simulink model "pendlib"  (Simulink 7.4)
settings: Solver=ode45  StartTime=0.0  StopTime=10.0  RelTol=1e-3
values from neighbouring files (symbols this model uses):
  Fscomp_neg = 0.16    [pendinit.m]
  Fscomp_pos = 0.16    [pendinit.m]
  g = 9.81    [pendinit.m]
  h = 0.01    [pendinit.m]
  J = 0.05    [pendinit.m]
  Jp = 0.0009    [pendinit.m]
  k1 = 0.058    [pendinit.m]
  k2 = 0.68    [pendinit.m]
  k360 = 0.3091    [pendinit.m]
  k4r = 2.56    [pendinit.m]
  k5r = 2.0    (= 2)    [pendinit.m]
  kdot360 = 3.76    [pendinit.m]
  ku = 1.40    (= 1.4)    [pendinit.m]
  l = l + 1    (= 1)    [asdf.m]    (also in pendinit.m = 0.413)
  M = 0.01    [pendinit.m]
  m = 0.02    [pendinit.m]
  offs1 = 0.7792    [pendinit.m]
  offs2 = 0    [pendinit.m]
  offs360 = 5.1763    [pendinit.m]
  offs4r = 0    [pendinit.m]
  offs5r = 0.0708    [pendinit.m]
  offsdot360 = -0.022    [pendinit.m]
  r = 0.235    [pendinit.m]
  w0 = 5.58    [pendinit.m]
  x0 = [0.1 0 0 0]'    [pendinit.m]
undefined symbols (not defined in the file or in its folder): DiscIntNeverNeededParam
libraries: simulink3 x5
settings Model: Creator=lincoln  LastModifiedBy=karl  ExtModeTrigMode=oneshot  ExtModeArmWhenConnect=off  ExtModeAutoUpdateStatusClock=off
settings DataIOCC: LimitDataPoints=off
settings OptimizationCC: BooleanDataType=off  InitFltsAndDblsToZero=on
settings DebuggingCC: SaveWithParameterizedLinksMsg=none  SignalResolutionControl=TryResolveAllWithWarning  SolverPrmCheckMsg=none  MultiTaskDSMMsg=warning  MultiTaskCondExecSysMsg=none  StrictBusMsg=None
settings HardwareCC: TargetUnknown=on
settings RTWCC: IncludeERTFirstTime=on
settings GRTTargetCC: TargetFcnLib=ansi_tfl_tmw.mat

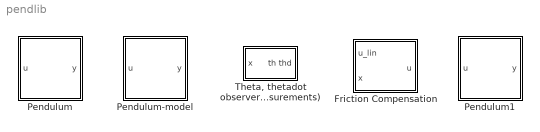
== system pendlib ==
  Friction Compensation : Subsystem  mask{khat=0}
      mask prompts: khat "k_hat"
  Pendulum : Subsystem
      mask Display: disp('Hardware')
  Pendulum-model : Subsystem
      mask Display: disp('Model')
  Pendulum1 : Subsystem
      mask Display: disp('Hardware\n Lab 2 Nonlin')
  "Theta, thetadot observer (for full 360 measurements)" : Subsystem

== system pendlib/Friction Compensation ==
  u_lin : Inport
  x : Inport  Port=2
  Friction model : Subsystem
  Selector : Selector  InputPortWidth=4  IndexOptions=Index vector (dialog)  Indices=4  OutputSizes=1
  u : Outport
  wires:
  Selector/1 -> Friction model/2(phidot)
  x/1 -> Selector/1
  u_lin/1 -> Friction model/1(u)
  Friction model/1(u_) -> u/1

== system pendlib/Pendulum ==
  u : Inport
  Hardware : Subsystem
  Safety net (switch off) : Subsystem
  Terminator : Terminator
  y : Outport  InitialOutput=0
  tag scope: u=global
  wires:
  Hardware/1(y) -> y/1
  Safety net (switch off)/1(u_out) -> [u], Hardware/1(u)
  u/1 -> Safety net (switch off)/1(u_in)
  [u] -> Terminator/1

== system pendlib/Pendulum-model ==
  u : Inport
  Pendulum Model : Subsystem
  Saturation : Saturate  UpperLimit=2  LowerLimit=-2
  Terminator : Terminator
  y : Outport  InitialOutput=0
  tag scope: u=global
  wires:
  Pendulum Model/1(x) -> y/1
  [u] -> Terminator/1
  u/1 -> Saturation/1
  Saturation/1 -> [u], Pendulum Model/1(u)

== system pendlib/Pendulum1 ==
  u : Inport
  Hardware : Subsystem
  Safety net (switch off) : Subsystem
  Terminator : Terminator
  y : Outport  InitialOutput=0
  tag scope: u=global
  wires:
  Hardware/1(y) -> y/1
  Safety net (switch off)/1(u_out) -> [u], Hardware/1(u)
  u/1 -> Safety net (switch off)/1(u_in)
  [u] -> Terminator/1

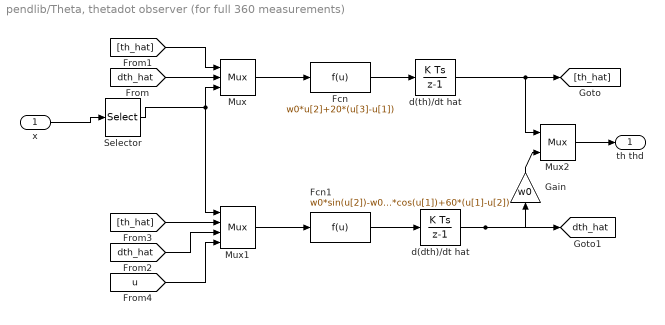
== system pendlib/Theta, thetadot observer (for full 360 measurements) ==
  x : Inport
  Fcn : Fcn  Expr=w0*u[2]+20*(u[3]-u[1])
  Fcn1 : Fcn  Expr=w0*sin(u[2])-w0*u[4]/g*cos(u[1])+60*(u[1]-u[2])
  Gain : Gain  Gain=w0  SaturateOnIntegerOverflow=on  OutDataTypeStr=Inherit: Same as input  ParamDataTypeStr=Inherit: Same as input
  Mux : Mux  Inputs=3
  Mux1 : Mux
  Mux2 : Mux  Inputs=2
  Selector : Selector  InputPortWidth=4  IndexOptions=Index vector (dialog)  Indices=1  OutputSizes=1
  d(dth)/dt hat : DiscreteIntegrator  SampleTime=h  ICPrevOutput=DiscIntNeverNeededParam  ICPrevScaledInput=DiscIntNeverNeededParam
  d(th)/dt hat : DiscreteIntegrator  InitialCondition=pi  SampleTime=h  ICPrevOutput=DiscIntNeverNeededParam  ICPrevScaledInput=DiscIntNeverNeededParam
  th thd : Outport
  tag scope: dth_hat=global
  wires:
  Mux/1 -> Fcn/1
  x/1 -> Selector/1
  Gain/1 -> Mux2/2
  d(dth)/dt hat/1 -> Gain/1, [dth_hat]
  [u] -> Mux1/4
  Fcn1/1 -> d(dth)/dt hat/1
  d(th)/dt hat/1 -> Mux2/1, [th_hat]
  Fcn/1 -> d(th)/dt hat/1
  [dth_hat] -> Mux1/3
  [th_hat] -> Mux1/2
  Mux1/1 -> Fcn1/1
  Mux2/1 -> th thd/1
  [dth_hat] -> Mux/2
  [th_hat] -> Mux/1
  Selector/1 -> Mux/3, Mux1/1

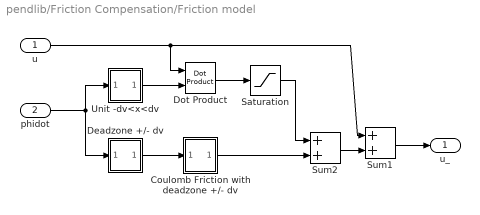
== system pendlib/Friction Compensation/Friction model ==
  u : Inport
  phidot : Inport  Port=2
  Coulomb Friction with deadzone +/- dv : Subsystem  mask{Fc_neg=khat, Fc_pos=khat, dv=0.06}
      mask prompts: Fc_neg "Coulomb Friction (Negative)"; Fc_pos "Coulomb Friction (Positive)"; dv "Deadzone width (Onesided)"
      mask Display:
      | plot([-1 0 0], [0 0 1], [0 0 1],[-1 0 0]);
      | plot([0.5 0.5 1],[0 0.5 0.5],[-0.5 -0.5 -1],[0 -0.5 -0.5]);
  Deadzone +/- dv : Subsystem  mask{vg=1, dv=0.06}
      mask prompts: vg "Gain"; dv "Deadzone width (Onesided)"
      mask init:
      | v_gain=vg;
      | d_v=dv;
      mask Display:
      | plot([-1 0 0], [0 0 1], [0 0 1],[-1 0 0]);
      | plot([0.5 0.5 1],[0 0.5 1],[-0.5 -0.5 -1],[0 -0.5 -1]);
  Dot Product : simulink3/Math/Dot Product  InputSameDT=on  DoSatur=off
  Saturation : Saturate  UpperLimit=khat  LowerLimit=-khat
  Sum1 : Sum  SaturateOnIntegerOverflow=on  InputSameDT=on  OutDataTypeStr=Inherit: Same as first input
  Sum2 : Sum  SaturateOnIntegerOverflow=on  InputSameDT=on  OutDataTypeStr=Inherit: Same as first input
  "Unit -dv<x<dv\t" : Subsystem  mask{dw=0.06}
      mask prompts: dw "Width (Onesided)"
      mask init:
      | d_w=dw;
      mask Display:
      | plot([-1 0 0], [0 0 1], [0 0 1],[-0.3 0 0]);
      | plot([-0.5 -0.5 0.5 0.5],[0 0.7 0.7 0])
  u_ : Outport  InitialOutput=0
  wires:
  phidot/1 -> "Unit -dv<x<dv\t"/1(In1), Deadzone +/- dv/1(In1)
  "Unit -dv<x<dv\t"/1(Out1) -> Dot Product/2
  Coulomb Friction with deadzone +/- dv/1(Out1) -> Sum2/2
  Dot Product/1 -> Saturation/1
  u/1 -> Dot Product/1, Sum1/1
  Saturation/1 -> Sum2/1
  Sum1/1 -> u_/1
  Deadzone +/- dv/1(Out1) -> Coulomb Friction with deadzone +/- dv/1(In1)
  Sum2/1 -> Sum1/2

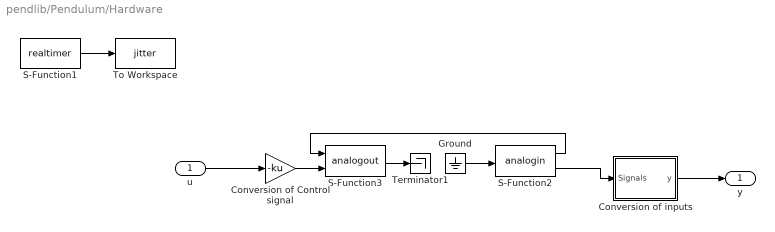
== system pendlib/Pendulum/Hardware ==
  u : Inport
  Conversion of Control signal : Gain  Gain=-ku  SaturateOnIntegerOverflow=on  OutDataTypeStr=Inherit: Same as input  ParamDataTypeStr=Inherit: Same as input
  Conversion of inputs : Subsystem
  Ground : Ground
  S-Function1 : S-Function  FunctionName=realtimer  Parameters=h  EnableBusSupport=off
  S-Function2 : S-Function  FunctionName=analogin  Parameters=h [0 0 1 1 2 2 3 3 4 4 5 5 6 6 7 7]  EnableBusSupport=off
  S-Function3 : S-Function  FunctionName=analogout  Parameters=h [0]  EnableBusSupport=off
  Terminator1 : Terminator
  To Workspace : ToWorkspace  VariableName=jitter  SampleTime=-1  SaveFormat=Array
  y : Outport
  wires:
  u/1 -> Conversion of Control signal/1
  Ground/1 -> S-Function2/1
  S-Function2/2 -> Conversion of inputs/1(Signals)
  S-Function3/1 -> Terminator1/1
  S-Function2/1 -> S-Function3/1
  Conversion of Control signal/1 -> S-Function3/2
  S-Function1/1 -> To Workspace/1
  Conversion of inputs/1(y) -> y/1

== system pendlib/Pendulum/Safety net (switch off) ==
  u_in : Inport
  Abs : Abs  SaturateOnIntegerOverflow=on
  Constant : Constant  Value=0
  Discrete Transfer Fcn : DiscreteTransferFcn  Numerator=[0.1]  Denominator=[1 -0.9]  SampleTime=h
  Relay : Relay  OnSwitchValue=3  OffSwitchValue=2
  Saturation1 : Saturate  UpperLimit=2  LowerLimit=-2
  Stop Simulation : Stop
  Switch : Switch  Threshold=0.5  SaturateOnIntegerOverflow=on  InputSameDT=on
  u_out : Outport
  wires:
  Discrete Transfer Fcn/1 -> Relay/1
  Relay/1 -> Stop Simulation/1, Switch/2
  Constant/1 -> Switch/1
  Abs/1 -> Discrete Transfer Fcn/1
  Switch/1 -> Saturation1/1
  Saturation1/1 -> u_out/1
  u_in/1 -> Switch/3, Abs/1

== system pendlib/Pendulum-model/Pendulum Model ==
  u : Inport
  "Friction Model Coulomb, Stic." : Subsystem
  Furuta pendulum : Subsystem  mask{l=l, M=M, Jp=Jp, r=r, J=J, m_w=m, g=g, x_0=x0}
      mask prompts: l "Pendulum Length"; M "Mass of Pendulum"; r "Length of Arm"; m_w "Mass of weight"
  Gain : Gain  Gain=g  SaturateOnIntegerOverflow=on  OutDataTypeStr=Inherit: Same as input  ParamDataTypeStr=Inherit: Same as input
  Sampling : Subsystem
  top-360 switching : Subsystem
  x : Outport  InitialOutput=0
  tag scope: phidot=global
  wires:
  top-360 switching/1(y_) -> x/1
  Sampling/1(x) -> top-360 switching/1(y)
  Furuta pendulum/1(angle) -> Sampling/1(Theta)
  Furuta pendulum/3(arm. ang.) -> Sampling/3(Phi)
  Furuta pendulum/2(angle vel.) -> Sampling/2(Thetadot)
  Furuta pendulum/4(arm. ang. vel.) -> Sampling/4(Phidot), [phidot]
  u/1 -> "Friction Model Coulomb, Stic."/1(u_)
  "Friction Model Coulomb, Stic."/1(u) -> Gain/1
  Gain/1 -> Furuta pendulum/1(u)

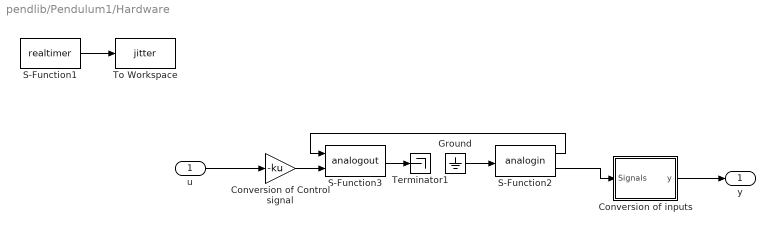
== system pendlib/Pendulum1/Hardware ==
  u : Inport
  Conversion of Control signal : Gain  Gain=-ku  SaturateOnIntegerOverflow=on  OutDataTypeStr=Inherit: Same as input  ParamDataTypeStr=Inherit: Same as input
  Conversion of inputs : Subsystem
  Ground : Ground
  S-Function1 : S-Function  FunctionName=realtimer  Parameters=h  EnableBusSupport=off
  S-Function2 : S-Function  FunctionName=analogin  Parameters=h [0 0 1 1 2 2 3 3 4 4 5 5 6 6 7 7]  EnableBusSupport=off
  S-Function3 : S-Function  FunctionName=analogout  Parameters=h [0]  EnableBusSupport=off
  Terminator1 : Terminator
  To Workspace : ToWorkspace  VariableName=jitter  SampleTime=-1  SaveFormat=Array
  y : Outport
  wires:
  u/1 -> Conversion of Control signal/1
  Ground/1 -> S-Function2/1
  S-Function2/2 -> Conversion of inputs/1(Signals)
  S-Function3/1 -> Terminator1/1
  S-Function2/1 -> S-Function3/1
  Conversion of Control signal/1 -> S-Function3/2
  S-Function1/1 -> To Workspace/1
  Conversion of inputs/1(y) -> y/1

== system pendlib/Pendulum1/Safety net (switch off) ==
  u_in : Inport
  Abs : Abs  SaturateOnIntegerOverflow=on
  Constant : Constant  Value=0
  Discrete Transfer Fcn : DiscreteTransferFcn  Numerator=[0.1]  Denominator=[1 -0.9]  SampleTime=h
  Relay : Relay  OnSwitchValue=3  OffSwitchValue=2
  Saturation1 : Saturate  UpperLimit=2  LowerLimit=-2
  Stop Simulation : Stop
  Switch : Switch  Threshold=0.5  SaturateOnIntegerOverflow=on  InputSameDT=on
  u_out : Outport
  wires:
  Discrete Transfer Fcn/1 -> Relay/1
  Relay/1 -> Stop Simulation/1, Switch/2
  Constant/1 -> Switch/1
  Abs/1 -> Discrete Transfer Fcn/1
  Switch/1 -> Saturation1/1
  Saturation1/1 -> u_out/1
  u_in/1 -> Switch/3, Abs/1

== system pendlib/Friction Compensation/Friction model/Coulomb Friction with deadzone +/- dv ==
  In1 : Inport
  Dead Zone : DeadZone  LowerValue=-dv  UpperValue=dv  SaturateOnIntegerOverflow=on
  Fcn : Fcn  Expr=(u<0)*u*Fc_neg+(u>0)*u*Fc_pos
  Sign : Signum
  Out1 : Outport  InitialOutput=0
  wires:
  Fcn/1 -> Out1/1
  Sign/1 -> Fcn/1
  Dead Zone/1 -> Sign/1
  In1/1 -> Dead Zone/1

== system pendlib/Friction Compensation/Friction model/Deadzone +/- dv ==
  In1 : Inport
  Constant : Constant  Value=d_v
  Dead Zone : DeadZone  LowerValue=-d_v  UpperValue=d_v  SaturateOnIntegerOverflow=on
  Dot Product : simulink3/Math/Dot Product  InputSameDT=on  DoSatur=off
  Gain : Gain  Gain=v_gain  SaturateOnIntegerOverflow=on  OutDataTypeStr=Inherit: Same as input  ParamDataTypeStr=Inherit: Same as input
  Sign : Signum
  Sum : Sum  SaturateOnIntegerOverflow=on  InputSameDT=on  OutDataTypeStr=Inherit: Same as first input
  Out1 : Outport  InitialOutput=0
  wires:
  Gain/1 -> Sum/1
  In1/1 -> Dead Zone/1
  Sign/1 -> Dot Product/1
  Dead Zone/1 -> Gain/1, Sign/1
  Constant/1 -> Dot Product/2
  Dot Product/1 -> Sum/2
  Sum/1 -> Out1/1

== system pendlib/Friction Compensation/Friction model/Unit -dv<x<dv	 ==
  In1 : Inport
  Abs : Abs  SaturateOnIntegerOverflow=on
  Constant : Constant
  Dead Zone : DeadZone  LowerValue=-d_w  UpperValue=d_w  SaturateOnIntegerOverflow=on
  Sign : Signum
  Sum1 : Sum  Inputs=+-  SaturateOnIntegerOverflow=on  InputSameDT=on  OutDataTypeStr=Inherit: Same as first input
  Out1 : Outport  InitialOutput=0
  wires:
  Dead Zone/1 -> Sign/1
  In1/1 -> Dead Zone/1
  Constant/1 -> Sum1/1
  Sum1/1 -> Out1/1
  Sign/1 -> Abs/1
  Abs/1 -> Sum1/2

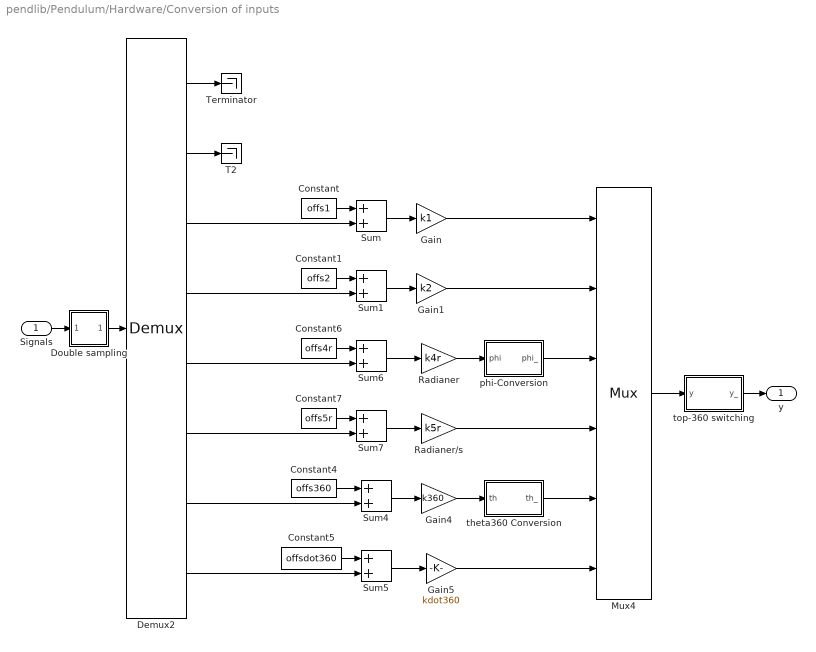
== system pendlib/Pendulum/Hardware/Conversion of inputs ==
  Signals : Inport
  Constant : Constant  Value=offs1
  Constant1 : Constant  Value=offs2
  Constant4 : Constant  Value=offs360
  Constant5 : Constant  Value=offsdot360
  Constant6 : Constant  Value=offs4r
  Constant7 : Constant  Value=offs5r
  Demux2 : Demux  Outputs=8
  Double sampling : Subsystem
  Gain : Gain  Gain=k1  SaturateOnIntegerOverflow=on  OutDataTypeStr=Inherit: Same as input  ParamDataTypeStr=Inherit: Same as input
  Gain1 : Gain  Gain=k2  SaturateOnIntegerOverflow=on  OutDataTypeStr=Inherit: Same as input  ParamDataTypeStr=Inherit: Same as input
  Gain4 : Gain  Gain=k360  SaturateOnIntegerOverflow=on  OutDataTypeStr=Inherit: Same as input  ParamDataTypeStr=Inherit: Same as input
  Gain5 : Gain  Gain=kdot360  SaturateOnIntegerOverflow=on  OutDataTypeStr=Inherit: Same as input  ParamDataTypeStr=Inherit: Same as input
  Mux4 : Mux  Inputs=6
  Radianer : Gain  Gain=k4r  SaturateOnIntegerOverflow=on  OutDataTypeStr=Inherit: Same as input  ParamDataTypeStr=Inherit: Same as input
  Radianer/s : Gain  Gain=k5r  SaturateOnIntegerOverflow=on  OutDataTypeStr=Inherit: Same as input  ParamDataTypeStr=Inherit: Same as input
  Sum{,1,4..7} (6 alike) : Sum  SaturateOnIntegerOverflow=on  InputSameDT=on  OutDataTypeStr=Inherit: Same as first input
  T2 : Terminator
  Terminator : Terminator
  phi-Conversion : Subsystem
  theta360 Conversion : Subsystem
  top-360 switching : Subsystem
  y : Outport  InitialOutput=0
  wires:
  Demux2/2 -> T2/1
  Demux2/1 -> Terminator/1
  Sum/1 -> Gain/1
  Constant/1 -> Sum/1
  Sum1/1 -> Gain1/1
  Constant1/1 -> Sum1/1
  Sum4/1 -> Gain4/1
  Sum5/1 -> Gain5/1
  Constant5/1 -> Sum5/1
  Sum6/1 -> Radianer/1
  Constant6/1 -> Sum6/1
  Radianer/1 -> phi-Conversion/1(phi)
  Sum7/1 -> Radianer/s/1
  Constant7/1 -> Sum7/1
  Mux4/1 -> top-360 switching/1(y)
  top-360 switching/1(y_) -> y/1
  Constant4/1 -> Sum4/1
  Demux2/5 -> Sum6/2
  Demux2/6 -> Sum7/2
  phi-Conversion/1(phi_) -> Mux4/3
  Radianer/s/1 -> Mux4/4
  theta360 Conversion/1(th_) -> Mux4/5
  Signals/1 -> Double sampling/1(In1)
  Double sampling/1(Out1) -> Demux2/1
  Gain4/1 -> theta360 Conversion/1(th)
  Gain5/1 -> Mux4/6
  Gain/1 -> Mux4/1
  Demux2/3 -> Sum/2
  Demux2/4 -> Sum1/2
  Demux2/7 -> Sum4/2
  Demux2/8 -> Sum5/2
  Gain1/1 -> Mux4/2

== system pendlib/Pendulum-model/Pendulum Model/Friction Model Coulomb, Stic. ==
  u_ : Inport
  Friction model : Subsystem
  u : Outport  InitialOutput=0
  wires:
  Friction model/1(u_) -> u/1
  [phidot] -> Friction model/2(phidot)
  u_/1 -> Friction model/1(u)

== system pendlib/Pendulum-model/Pendulum Model/Furuta pendulum ==
  u : Inport
  Demux : Demux
  S-Function1 : S-Function  FunctionName=furuta  Parameters=l, M, Jp, r, J, m_w, g, x_0  EnableBusSupport=off
  angle : Outport  InitialOutput=0
  angle vel. : Outport  Port=2  InitialOutput=0
  arm. ang. : Outport  Port=3  InitialOutput=0
  arm. ang. vel. : Outport  Port=4  InitialOutput=0
  wires:
  Demux/4 -> arm. ang. vel./1
  Demux/3 -> arm. ang./1
  u/1 -> S-Function1/1
  Demux/2 -> angle vel./1
  Demux/1 -> angle/1
  S-Function1/1 -> Demux/1

== system pendlib/Pendulum-model/Pendulum Model/Sampling ==
  Theta : Inport
  Thetadot : Inport  Port=2
  Phi : Inport  Port=3
  Phidot : Inport  Port=4
  Demux : Demux  Outputs=[3 1]
  Mux : Mux
  Mux1 : Mux  Inputs=2
  Zero-Order Hold5 : ZeroOrderHold  SampleTime=h
  x : Outport  InitialOutput=0
  wires:
  Demux/2 -> Mux1/2
  Theta/1 -> Mux/1
  Thetadot/1 -> Mux/2
  Phi/1 -> Mux/3
  Phidot/1 -> Mux/4
  Mux/1 -> Zero-Order Hold5/1
  Zero-Order Hold5/1 -> Demux/1
  Mux1/1 -> x/1
  Demux/1 -> Mux1/1

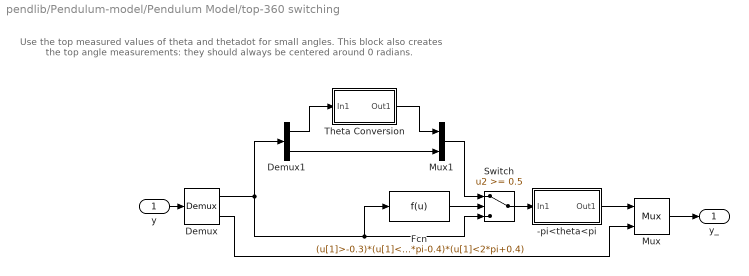
== system pendlib/Pendulum-model/Pendulum Model/top-360 switching ==
  note: Use the top measured values of
      | theta and thetadot for small angles.
      | This block also creates the top angle
      | measurements: they should always be
      | centered around 0 radians.
  y : Inport
  -pi<theta<pi : Subsystem
  Demux : Demux  Outputs=[2 2]
  Demux1 : Demux  Outputs=2
  Fcn : Fcn  Expr=(u[1]>-0.3)*(u[1]<0.4)+(u[1]>2*pi-0.4)*(u[1]<2*pi+0.4)
  Mux : Mux  Inputs=2
  Mux1 : Mux  Inputs=2
  Switch : Switch  Threshold=0.5  SaturateOnIntegerOverflow=on  InputSameDT=on
  Theta Conversion : Subsystem
  y_ : Outport
  wires:
  Mux1/1 -> Switch/1
  Demux1/2 -> Mux1/2
  Demux1/1 -> Theta Conversion/1(In1)
  Demux/1 -> Fcn/1, Switch/3, Demux1/1
  Demux/2 -> Mux/2
  y/1 -> Demux/1
  Mux/1 -> y_/1
  Fcn/1 -> Switch/2
  Theta Conversion/1(Out1) -> Mux1/1
  Switch/1 -> -pi<theta<pi/1(In1)
  -pi<theta<pi/1(Out1) -> Mux/1

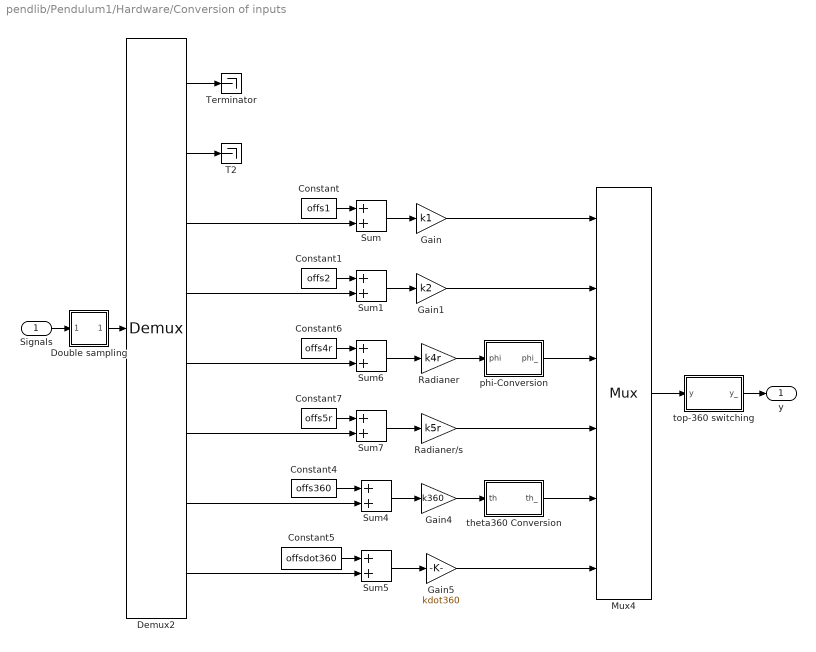
== system pendlib/Pendulum1/Hardware/Conversion of inputs ==
  Signals : Inport
  Constant : Constant  Value=offs1
  Constant1 : Constant  Value=offs2
  Constant4 : Constant  Value=offs360
  Constant5 : Constant  Value=offsdot360
  Constant6 : Constant  Value=offs4r
  Constant7 : Constant  Value=offs5r
  Demux2 : Demux  Outputs=8
  Double sampling : Subsystem
  Gain : Gain  Gain=k1  SaturateOnIntegerOverflow=on  OutDataTypeStr=Inherit: Same as input  ParamDataTypeStr=Inherit: Same as input
  Gain1 : Gain  Gain=k2  SaturateOnIntegerOverflow=on  OutDataTypeStr=Inherit: Same as input  ParamDataTypeStr=Inherit: Same as input
  Gain4 : Gain  Gain=k360  SaturateOnIntegerOverflow=on  OutDataTypeStr=Inherit: Same as input  ParamDataTypeStr=Inherit: Same as input
  Gain5 : Gain  Gain=kdot360  SaturateOnIntegerOverflow=on  OutDataTypeStr=Inherit: Same as input  ParamDataTypeStr=Inherit: Same as input
  Mux4 : Mux  Inputs=6
  Radianer : Gain  Gain=k4r  SaturateOnIntegerOverflow=on  OutDataTypeStr=Inherit: Same as input  ParamDataTypeStr=Inherit: Same as input
  Radianer/s : Gain  Gain=k5r  SaturateOnIntegerOverflow=on  OutDataTypeStr=Inherit: Same as input  ParamDataTypeStr=Inherit: Same as input
  Sum{,1,4..7} (6 alike) : Sum  SaturateOnIntegerOverflow=on  InputSameDT=on  OutDataTypeStr=Inherit: Same as first input
  T2 : Terminator
  Terminator : Terminator
  phi-Conversion : Subsystem
  theta360 Conversion : Subsystem
  top-360 switching : Subsystem
  y : Outport  InitialOutput=0
  wires:
  Demux2/2 -> T2/1
  Demux2/1 -> Terminator/1
  Sum/1 -> Gain/1
  Constant/1 -> Sum/1
  Sum1/1 -> Gain1/1
  Constant1/1 -> Sum1/1
  Sum4/1 -> Gain4/1
  Sum5/1 -> Gain5/1
  Constant5/1 -> Sum5/1
  Sum6/1 -> Radianer/1
  Constant6/1 -> Sum6/1
  Radianer/1 -> phi-Conversion/1(phi)
  Sum7/1 -> Radianer/s/1
  Constant7/1 -> Sum7/1
  Mux4/1 -> top-360 switching/1(y)
  top-360 switching/1(y_) -> y/1
  Constant4/1 -> Sum4/1
  Demux2/5 -> Sum6/2
  Demux2/6 -> Sum7/2
  phi-Conversion/1(phi_) -> Mux4/3
  Radianer/s/1 -> Mux4/4
  theta360 Conversion/1(th_) -> Mux4/5
  Signals/1 -> Double sampling/1(In1)
  Double sampling/1(Out1) -> Demux2/1
  Gain4/1 -> theta360 Conversion/1(th)
  Gain5/1 -> Mux4/6
  Gain/1 -> Mux4/1
  Demux2/3 -> Sum/2
  Demux2/4 -> Sum1/2
  Demux2/7 -> Sum4/2
  Demux2/8 -> Sum5/2
  Gain1/1 -> Mux4/2

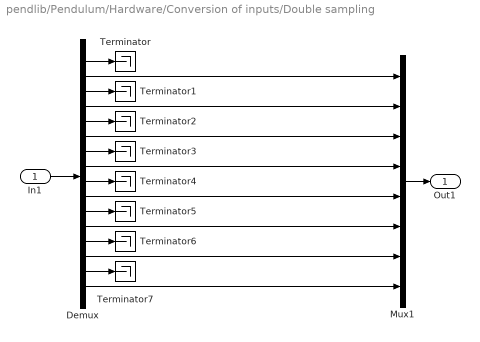
== system pendlib/Pendulum/Hardware/Conversion of inputs/Double sampling ==
  In1 : Inport
  Demux : Demux  Outputs=16
  Mux1 : Mux  Inputs=8
  Terminator{,1..7} (8 alike) : Terminator
  Out1 : Outport
  wires:
  Demux/7 -> Terminator3/1
  Demux/9 -> Terminator4/1
  Demux/11 -> Terminator5/1
  Demux/13 -> Terminator6/1
  Demux/15 -> Terminator7/1
  Demux/5 -> Terminator2/1
  Demux/3 -> Terminator1/1
  Demux/1 -> Terminator/1
  In1/1 -> Demux/1
  Demux/2 -> Mux1/1
  Mux1/1 -> Out1/1
  Demux/4 -> Mux1/2
  Demux/6 -> Mux1/3
  Demux/8 -> Mux1/4
  Demux/10 -> Mux1/5
  Demux/12 -> Mux1/6
  Demux/14 -> Mux1/7
  Demux/16 -> Mux1/8

== system pendlib/Pendulum/Hardware/Conversion of inputs/phi-Conversion ==
  note: This block deals with the discontinious nature
      | of the phi signal. The offset is kept in the integrator.
  phi : Inport
  Diff : DiscreteTransferFcn  Numerator=[1 -1]  Denominator=[1 0]  SampleTime=h
  Extended Deadzone : Subsystem  mask{vg=1, dv=0.5}
      mask prompts: vg "Gain"; dv "Deadzone width"
      mask init:
      | v_gain=vg;
      | d_v=dv;
      mask Display:
      | plot([-1 0 0], [0 0 1], [0 0 1],[-1 0 0]);
      | plot([0.5 0.5 1],[0 0.5 1],[-0.5 -0.5 -1],[0 -0.5 -1]);
  Gain1 : Gain  Gain=-1  SaturateOnIntegerOverflow=on  OutDataTypeStr=Inherit: Same as input  ParamDataTypeStr=Inherit: Same as input
  Integrate : DiscreteTransferFcn  Denominator=[1 -1]  SampleTime=h
  Sum2 : Sum  SaturateOnIntegerOverflow=on  InputSameDT=on  OutDataTypeStr=Inherit: Same as first input
  Sum3 : Sum  SaturateOnIntegerOverflow=on  InputSameDT=on  OutDataTypeStr=Inherit: Same as first input
  phi_ : Outport
  wires:
  Sum2/1 -> Gain1/1
  phi/1 -> Diff/1, Sum3/2
  Gain1/1 -> Sum3/1
  Integrate/1 -> Sum2/2
  Extended Deadzone/1(Out1) -> Integrate/1, Sum2/1
  Sum3/1 -> phi_/1
  Diff/1 -> Extended Deadzone/1(In1)

== system pendlib/Pendulum/Hardware/Conversion of inputs/theta360 Conversion ==
  note: The measure of Theta is discontinous and must hereby
      | be modifyed in order to give a reasonable continous signal.
  th : Inport
  Fcn : Fcn  Expr=((u[1]-u[2])>2)*(-2*pi)+((u[1]-u[2])<-2)*(2*pi)
  Last sample : UnitDelay  X0=pi  SampleTime=h
  Mux : Mux  Inputs=2
  Offset : Subsystem
  Scope2 : Scope
      settings: TimeRange=25  YMin=-0.4  YMax=0.05
  Spike Filter6 : Subsystem
  Sum3 : Sum  SaturateOnIntegerOverflow=on  InputSameDT=on  OutDataTypeStr=Inherit: Same as first input
  th_ : Outport
  wires:
  Mux/1 -> Fcn/1
  th/1 -> Last sample/1, Mux/1, Sum3/1
  Last sample/1 -> Mux/2
  Fcn/1 -> Offset/1(In1)
  Offset/1(Out1) -> Sum3/2
  Sum3/1 -> Spike Filter6/1(x)
  Spike Filter6/1(x_) -> th_/1, Scope2/1

== system pendlib/Pendulum/Hardware/Conversion of inputs/top-360 switching ==
  note: Use the top measured values of
      | theta and thetadot for small angles
  y : Inport
  Demux : Demux  Outputs=[2 2 2]
  Fcn : Fcn  Expr=(u[1]>-0.5)*(u[1]<0.5)+(u[1]>2*pi-0.5)*(u[1]<2*pi+0.5)
  Mux : Mux  Inputs=2
  Switch : Switch  Threshold=0.5  SaturateOnIntegerOverflow=on  InputSameDT=on
  y_ : Outport
  wires:
  y/1 -> Demux/1
  Demux/2 -> Mux/2
  Demux/1 -> Switch/1
  Demux/3 -> Switch/3, Fcn/1
  Switch/1 -> Mux/1
  Fcn/1 -> Switch/2
  Mux/1 -> y_/1

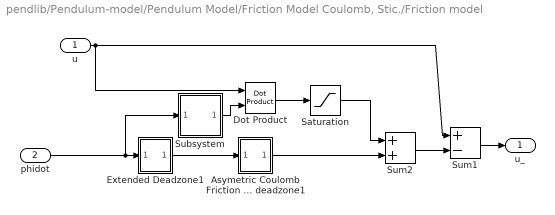
== system pendlib/Pendulum-model/Pendulum Model/Friction Model Coulomb, Stic./Friction model ==
  u : Inport
  phidot : Inport  Port=2
  Asymetric Coulomb Friction with deadzone1 : Subsystem  mask{Fc_neg=Fscomp_neg, Fc_pos=Fscomp_pos, dv=0.04}
      mask prompts: Fc_neg "Coulomb Friction (Negative)"; Fc_pos "Coulomb Friction (Positive)"; dv "Deadzone width (Onesided)"
      mask Display:
      | plot([-1 0 0], [0 0 1], [0 0 1],[-1 0 0]);
      | plot([0.5 0.5 1],[0 0.5 0.5],[-0.5 -0.5 -1],[0 -0.5 -0.5]);
  Dot Product : simulink3/Math/Dot Product  InputSameDT=on  DoSatur=off
  Extended Deadzone1 : Subsystem  mask{vg=1, dv=0.04}
      mask prompts: vg "Gain"; dv "Deadzone width (Onesided)"
      mask init:
      | v_gain=vg;
      | d_v=dv;
      mask Display:
      | plot([-1 0 0], [0 0 1], [0 0 1],[-1 0 0]);
      | plot([0.5 0.5 1],[0 0.5 1],[-0.5 -0.5 -1],[0 -0.5 -1]);
  Saturation : Saturate  UpperLimit=Fscomp_pos  LowerLimit=-Fscomp_neg
  Subsystem : Subsystem  mask{dw=0.04}
      mask prompts: dw "Width (Onesided)"
      mask init:
      | d_w=dw;
      mask Display:
      | plot([-1 0 0], [0 0 1], [0 0 1],[-0.3 0 0]);
      | plot([-0.5 -0.5 0.5 0.5],[0 0.7 0.7 0])
  Sum1 : Sum  Inputs=+-  SaturateOnIntegerOverflow=on  InputSameDT=on  OutDataTypeStr=Inherit: Same as first input
  Sum2 : Sum  SaturateOnIntegerOverflow=on  InputSameDT=on  OutDataTypeStr=Inherit: Same as first input
  u_ : Outport  InitialOutput=0
  wires:
  Asymetric Coulomb Friction with deadzone1/1(Out1) -> Sum2/2
  Sum2/1 -> Sum1/2
  u/1 -> Sum1/1, Dot Product/1
  Dot Product/1 -> Saturation/1
  Subsystem/1(Out1) -> Dot Product/2
  Extended Deadzone1/1(Out1) -> Asymetric Coulomb Friction with deadzone1/1(In1)
  Sum1/1 -> u_/1
  phidot/1 -> Subsystem/1(In1), Extended Deadzone1/1(In1)
  Saturation/1 -> Sum2/1

== system pendlib/Pendulum-model/Pendulum Model/top-360 switching/-pi<theta<pi ==
  In1 : Inport
  Constant : Constant  Value=2*pi
  Constant1 : Constant  Value=pi
  Demux : Demux  Outputs=2
  Math Function : Math  Operator=mod  SaturateOnIntegerOverflow=on
  Mux : Mux  Inputs=2
  Product : Product  SaturateOnIntegerOverflow=on  RndMeth=Zero  InputSameDT=on  OutDataTypeStr=Inherit: Same as first input
  Relational Operator : RelationalOperator  InputSameDT=on
  Sum : Sum  Inputs=|+-  SaturateOnIntegerOverflow=on  InputSameDT=on  OutDataTypeStr=Inherit: Same as first input
  Out1 : Outport
  wires:
  Constant/1 -> Math Function/2, Product/2
  Math Function/1 -> Sum/1, Relational Operator/1
  Constant1/1 -> Relational Operator/2
  Relational Operator/1 -> Product/1
  Product/1 -> Sum/2
  In1/1 -> Demux/1
  Demux/1 -> Math Function/1
  Sum/1 -> Mux/1
  Mux/1 -> Out1/1
  Demux/2 -> Mux/2

== system pendlib/Pendulum-model/Pendulum Model/top-360 switching/Theta Conversion ==
  In1 : Inport
  Fcn1 : Fcn  Expr=(u[1]-u[2])*2*pi-pi
  Fcn2 : Fcn  Expr=u/(2*pi)-1/2
  Mux : Mux  Inputs=2
  Rounding Function : Rounding
  Out1 : Outport  InitialOutput=0
  wires:
  Rounding Function/1 -> Mux/2
  Fcn2/1 -> Rounding Function/1, Mux/1
  Mux/1 -> Fcn1/1
  Fcn1/1 -> Out1/1
  In1/1 -> Fcn2/1

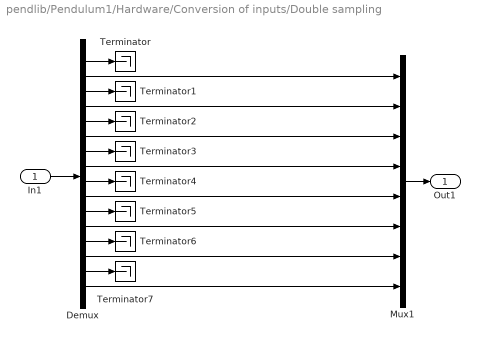
== system pendlib/Pendulum1/Hardware/Conversion of inputs/Double sampling ==
  In1 : Inport
  Demux : Demux  Outputs=16
  Mux1 : Mux  Inputs=8
  Terminator{,1..7} (8 alike) : Terminator
  Out1 : Outport
  wires:
  Demux/7 -> Terminator3/1
  Demux/9 -> Terminator4/1
  Demux/11 -> Terminator5/1
  Demux/13 -> Terminator6/1
  Demux/15 -> Terminator7/1
  Demux/5 -> Terminator2/1
  Demux/3 -> Terminator1/1
  Demux/1 -> Terminator/1
  In1/1 -> Demux/1
  Demux/2 -> Mux1/1
  Mux1/1 -> Out1/1
  Demux/4 -> Mux1/2
  Demux/6 -> Mux1/3
  Demux/8 -> Mux1/4
  Demux/10 -> Mux1/5
  Demux/12 -> Mux1/6
  Demux/14 -> Mux1/7
  Demux/16 -> Mux1/8

== system pendlib/Pendulum1/Hardware/Conversion of inputs/phi-Conversion ==
  note: This block deals with the discontinious nature
      | of the phi signal. The offset is kept in the integrator.
  phi : Inport
  Diff : DiscreteTransferFcn  Numerator=[1 -1]  Denominator=[1 0]  SampleTime=h
  Extended Deadzone : Subsystem  mask{vg=1, dv=0.5}
      mask prompts: vg "Gain"; dv "Deadzone width"
      mask init:
      | v_gain=vg;
      | d_v=dv;
      mask Display:
      | plot([-1 0 0], [0 0 1], [0 0 1],[-1 0 0]);
      | plot([0.5 0.5 1],[0 0.5 1],[-0.5 -0.5 -1],[0 -0.5 -1]);
  Gain1 : Gain  Gain=-1  SaturateOnIntegerOverflow=on  OutDataTypeStr=Inherit: Same as input  ParamDataTypeStr=Inherit: Same as input
  Integrate : DiscreteTransferFcn  Denominator=[1 -1]  SampleTime=h
  Sum2 : Sum  SaturateOnIntegerOverflow=on  InputSameDT=on  OutDataTypeStr=Inherit: Same as first input
  Sum3 : Sum  SaturateOnIntegerOverflow=on  InputSameDT=on  OutDataTypeStr=Inherit: Same as first input
  phi_ : Outport
  wires:
  Sum2/1 -> Gain1/1
  phi/1 -> Diff/1, Sum3/2
  Gain1/1 -> Sum3/1
  Integrate/1 -> Sum2/2
  Extended Deadzone/1(Out1) -> Integrate/1, Sum2/1
  Sum3/1 -> phi_/1
  Diff/1 -> Extended Deadzone/1(In1)

== system pendlib/Pendulum1/Hardware/Conversion of inputs/theta360 Conversion ==
  note: The measure of Theta is discontinous and must hereby
      | be modifyed in order to give a reasonable continous signal.
  th : Inport
  Fcn : Fcn  Expr=((u[1]-u[2])>2)*(-2*pi)+((u[1]-u[2])<-2)*(2*pi)
  Last sample : UnitDelay  X0=pi  SampleTime=h
  Mux : Mux  Inputs=2
  Offset : Subsystem
  Scope2 : Scope
      settings: TimeRange=25  YMin=-0.4  YMax=0.05
  Spike Filter6 : Subsystem
  Sum3 : Sum  SaturateOnIntegerOverflow=on  InputSameDT=on  OutDataTypeStr=Inherit: Same as first input
  th_ : Outport
  wires:
  Mux/1 -> Fcn/1
  th/1 -> Last sample/1, Mux/1, Sum3/1
  Last sample/1 -> Mux/2
  Fcn/1 -> Offset/1(In1)
  Offset/1(Out1) -> Sum3/2
  Sum3/1 -> Spike Filter6/1(x)
  Spike Filter6/1(x_) -> th_/1, Scope2/1

== system pendlib/Pendulum1/Hardware/Conversion of inputs/top-360 switching ==
  note: Use the top measured values of
      | theta and thetadot for small angles
  y : Inport
  Demux : Demux  Outputs=[2 2 2]
  Fcn : Fcn  Expr=(u[1]>-0.5)*(u[1]<0.5)+(u[1]>2*pi-0.5)*(u[1]<2*pi+0.5)
  ModTheta : Subsystem
  Mux : Mux  Inputs=2
  Scope1 : Scope
      settings: YMin=-4  YMax=7  SaveName=ScopeData3
  Switch : Switch  Threshold=0.5  SaturateOnIntegerOverflow=on  InputSameDT=on
  y_ : Outport
  wires:
  Switch/1 -> Mux/1
  ModTheta/1(xMod) -> Fcn/1, Switch/3
  Demux/3 -> ModTheta/1(x)
  y/1 -> Demux/1
  Demux/2 -> Mux/2
  Demux/1 -> Scope1/1, Switch/1
  Fcn/1 -> Switch/2
  Mux/1 -> y_/1

== system pendlib/Pendulum/Hardware/Conversion of inputs/phi-Conversion/Extended Deadzone ==
  In1 : Inport
  Constant : Constant  Value=d_v
  Dead Zone : DeadZone  LowerValue=-d_v  UpperValue=d_v  SaturateOnIntegerOverflow=on
  Dot Product : simulink3/Math/Dot Product  InputSameDT=on  DoSatur=off
  Gain : Gain  Gain=v_gain  SaturateOnIntegerOverflow=on  OutDataTypeStr=Inherit: Same as input  ParamDataTypeStr=Inherit: Same as input
  Sign : Signum
  Sum : Sum  SaturateOnIntegerOverflow=on  InputSameDT=on  OutDataTypeStr=Inherit: Same as first input
  Out1 : Outport  InitialOutput=0
  wires:
  Sum/1 -> Out1/1
  Dot Product/1 -> Sum/2
  Constant/1 -> Dot Product/2
  Dead Zone/1 -> Sign/1, Gain/1
  Sign/1 -> Dot Product/1
  In1/1 -> Dead Zone/1
  Gain/1 -> Sum/1

== system pendlib/Pendulum/Hardware/Conversion of inputs/theta360 Conversion/Offset ==
  note: Make sure only one
      | trig per lap.
  In1 : Inport
  Fcn : Fcn  Expr=(abs(u[1]+u[2])>8)*0+(abs(u[1]+u[2])<8)*u[1]
  Integrate : DiscreteTransferFcn  Denominator=[1 -1]  SampleTime=h
  Last offset : UnitDelay  X0=pi  SampleTime=h
  Mux : Mux  Inputs=2
  Out1 : Outport  InitialOutput=0
  wires:
  Mux/1 -> Fcn/1
  In1/1 -> Mux/1, Last offset/1
  Last offset/1 -> Mux/2
  Fcn/1 -> Integrate/1
  Integrate/1 -> Out1/1

== system pendlib/Pendulum/Hardware/Conversion of inputs/theta360 Conversion/Spike Filter6 ==
  x : Inport
  Fcn : Fcn  Expr=(abs(u[1]-u[2])<0.5)*u[1]+(abs(u[1]-u[2])>0.5)*u[3]
  Last Chosen : UnitDelay  X0=pi  SampleTime=h
  Last sample : UnitDelay  X0=pi  SampleTime=h
  Mux : Mux  Inputs=3
  Scope1 : Scope
      settings: YMin=0  YMax=11
  Scope2 : Scope
      settings: YMin=9  YMax=9.9
  x_ : Outport
  wires:
  Last Chosen/1 -> Mux/3
  Last sample/1 -> Mux/2
  x/1 -> Last sample/1, Mux/1
  Fcn/1 -> x_/1, Scope1/1, Last Chosen/1
  Mux/1 -> Fcn/1, Scope2/1

== system pendlib/Pendulum-model/Pendulum Model/Friction Model Coulomb, Stic./Friction model/Asymetric Coulomb Friction with deadzone1 ==
  In1 : Inport
  Dead Zone : DeadZone  LowerValue=-dv  UpperValue=dv  SaturateOnIntegerOverflow=on
  Fcn : Fcn  Expr=(u<0)*u*Fc_neg+(u>0)*u*Fc_pos
  Sign : Signum
  Out1 : Outport  InitialOutput=0
  wires:
  In1/1 -> Dead Zone/1
  Dead Zone/1 -> Sign/1
  Sign/1 -> Fcn/1
  Fcn/1 -> Out1/1

== system pendlib/Pendulum-model/Pendulum Model/Friction Model Coulomb, Stic./Friction model/Extended Deadzone1 ==
  In1 : Inport
  Constant : Constant  Value=d_v
  Dead Zone : DeadZone  LowerValue=-d_v  UpperValue=d_v  SaturateOnIntegerOverflow=on
  Dot Product : simulink3/Math/Dot Product  InputSameDT=on  DoSatur=off
  Gain : Gain  Gain=v_gain  SaturateOnIntegerOverflow=on  OutDataTypeStr=Inherit: Same as input  ParamDataTypeStr=Inherit: Same as input
  Sign : Signum
  Sum : Sum  SaturateOnIntegerOverflow=on  InputSameDT=on  OutDataTypeStr=Inherit: Same as first input
  Out1 : Outport  InitialOutput=0
  wires:
  Sum/1 -> Out1/1
  Dot Product/1 -> Sum/2
  Constant/1 -> Dot Product/2
  Dead Zone/1 -> Sign/1, Gain/1
  Sign/1 -> Dot Product/1
  In1/1 -> Dead Zone/1
  Gain/1 -> Sum/1

== system pendlib/Pendulum-model/Pendulum Model/Friction Model Coulomb, Stic./Friction model/Subsystem ==
  In1 : Inport
  Abs : Abs  SaturateOnIntegerOverflow=on
  Constant : Constant
  Dead Zone : DeadZone  LowerValue=-d_w  UpperValue=d_w  SaturateOnIntegerOverflow=on
  Sign : Signum
  Sum1 : Sum  Inputs=+-  SaturateOnIntegerOverflow=on  InputSameDT=on  OutDataTypeStr=Inherit: Same as first input
  Out1 : Outport  InitialOutput=0
  wires:
  Abs/1 -> Sum1/2
  Sign/1 -> Abs/1
  Sum1/1 -> Out1/1
  Constant/1 -> Sum1/1
  In1/1 -> Dead Zone/1
  Dead Zone/1 -> Sign/1

== system pendlib/Pendulum1/Hardware/Conversion of inputs/phi-Conversion/Extended Deadzone ==
  In1 : Inport
  Constant : Constant  Value=d_v
  Dead Zone : DeadZone  LowerValue=-d_v  UpperValue=d_v  SaturateOnIntegerOverflow=on
  Dot Product : DotProduct  OutDataType=fixdt(1, 16)  OutScaling=2^-10  InputSameDT=on  OutDataTypeStr=Inherit: Inherit via internal rule
  Gain : Gain  Gain=v_gain  SaturateOnIntegerOverflow=on  OutDataTypeStr=Inherit: Same as input  ParamDataTypeStr=Inherit: Same as input
  Sign : Signum
  Sum : Sum  SaturateOnIntegerOverflow=on  InputSameDT=on  OutDataTypeStr=Inherit: Same as first input
  Out1 : Outport  InitialOutput=0
  wires:
  Sum/1 -> Out1/1
  Dot Product/1 -> Sum/2
  Constant/1 -> Dot Product/2
  Dead Zone/1 -> Sign/1, Gain/1
  Sign/1 -> Dot Product/1
  In1/1 -> Dead Zone/1
  Gain/1 -> Sum/1

== system pendlib/Pendulum1/Hardware/Conversion of inputs/theta360 Conversion/Offset ==
  note: Make sure only one
      | trig per lap.
  In1 : Inport
  Fcn : Fcn  Expr=(abs(u[1]+u[2])>8)*0+(abs(u[1]+u[2])<8)*u[1]
  Integrate : DiscreteTransferFcn  Denominator=[1 -1]  SampleTime=h
  Last offset : UnitDelay  X0=pi  SampleTime=h
  Mux : Mux  Inputs=2
  Out1 : Outport  InitialOutput=0
  wires:
  Mux/1 -> Fcn/1
  In1/1 -> Mux/1, Last offset/1
  Last offset/1 -> Mux/2
  Fcn/1 -> Integrate/1
  Integrate/1 -> Out1/1

== system pendlib/Pendulum1/Hardware/Conversion of inputs/theta360 Conversion/Spike Filter6 ==
  x : Inport
  Fcn : Fcn  Expr=(abs(u[1]-u[2])<0.5)*u[1]+(abs(u[1]-u[2])>0.5)*u[3]
  Last Chosen : UnitDelay  X0=pi  SampleTime=h
  Last sample : UnitDelay  X0=pi  SampleTime=h
  Mux : Mux  Inputs=3
  Scope1 : Scope
      settings: YMin=0  YMax=11
  Scope2 : Scope
      settings: YMin=9  YMax=9.9
  x_ : Outport
  wires:
  Last Chosen/1 -> Mux/3
  Last sample/1 -> Mux/2
  x/1 -> Last sample/1, Mux/1
  Fcn/1 -> x_/1, Scope1/1, Last Chosen/1
  Mux/1 -> Fcn/1, Scope2/1

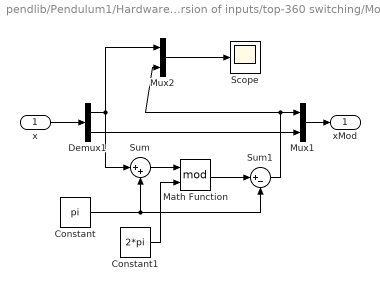
== system pendlib/Pendulum1/Hardware/Conversion of inputs/top-360 switching/ModTheta ==
  x : Inport
  Constant : Constant  Value=pi  OutDataType=fixdt(1, 16)  OutScaling=2^0
  Constant1 : Constant  Value=2*pi  OutDataType=fixdt(1, 16)  OutScaling=2^0
  Demux1 : Demux  Outputs=2
  Math Function : Math  Operator=mod  OutDataType=fixdt(1, 16)  OutScaling=2^0  SaturateOnIntegerOverflow=on
  Mux1 : Mux  Inputs=2
  Mux2 : Mux  Inputs=2
  Scope : Scope
      settings: YMin=-4  YMax=7  SaveName=ScopeData2
  Sum : Sum  Inputs=|++  OutDataType=fixdt(1, 16)  OutScaling=2^0
  Sum1 : Sum  Inputs=|+-  OutDataType=fixdt(1, 16)  OutScaling=2^0
  xMod : Outport
  wires:
  Mux1/1 -> xMod/1
  x/1 -> Demux1/1
  Sum1/1 -> Mux2/2, Mux1/1
  Math Function/1 -> Sum1/1
  Constant1/1 -> Math Function/2
  Sum/1 -> Math Function/1
  Demux1/2 -> Mux1/2
  Constant/1 -> Sum1/2, Sum/2
  Mux2/1 -> Scope/1
  Demux1/1 -> Sum/1, Mux2/1
